simulink model "Wiper_System"  (R2018a)
settings: Solver=FixedStepDiscrete  StartTime=0.0  StopTime=10.0  FixedStep=0.01  RelTol=1e-3
settings Model: Creator=Choaib ELMADI  LastModifiedBy=Choaib ELMADI

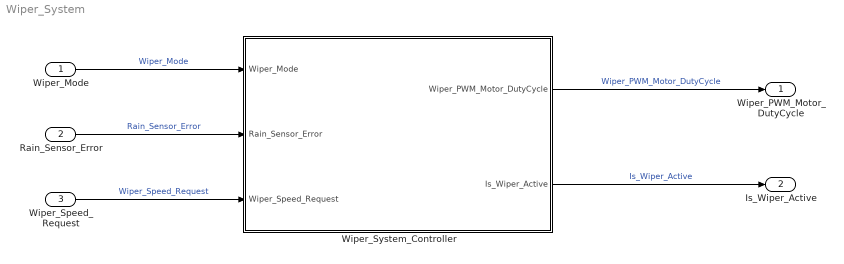
== system Wiper_System ==
  Wiper_Mode : Inport  OutMin=0  OutMax=3  OutDataTypeStr=double
  Rain_Sensor_Error : Inport  Port=2  OutMin=0  OutMax=1  OutDataTypeStr=double
  Wiper_Speed_Request : Inport  Port=3  OutMin=0  OutMax=7  OutDataTypeStr=double
  Wiper_System_Controller : Subsystem
  Wiper_PWM_Motor_DutyCycle : Outport  OutMin=0  OutMax=1  OutDataTypeStr=double
  Is_Wiper_Active : Outport  Port=2  OutMin=0  OutMax=1  OutDataTypeStr=double
  wires:
  Wiper_Mode/1 -> Wiper_System_Controller/1(Wiper_Mode)  "Wiper_Mode"
  Rain_Sensor_Error/1 -> Wiper_System_Controller/2(Rain_Sensor_Error)  "Rain_Sensor_Error"
  Wiper_Speed_Request/1 -> Wiper_System_Controller/3(Wiper_Speed_Request)  "Wiper_Speed_Request"
  Wiper_System_Controller/1(Wiper_PWM_Motor_DutyCycle) -> Wiper_PWM_Motor_DutyCycle/1  "Wiper_PWM_Motor_DutyCycle"
  Wiper_System_Controller/2(Is_Wiper_Active) -> Is_Wiper_Active/1  "Is_Wiper_Active"

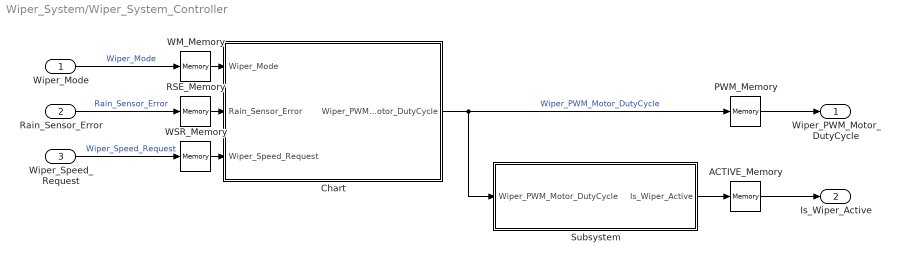
== system Wiper_System/Wiper_System_Controller ==
  Wiper_Mode : Inport
  Rain_Sensor_Error : Inport  Port=2
  Wiper_Speed_Request : Inport  Port=3
  ACTIVE_Memory : Memory
  Chart : Stateflow chart  TreatAsAtomicUnit=on
  PWM_Memory : Memory
  RSE_Memory : Memory
  Subsystem : Subsystem
  WM_Memory : Memory
  WSR_Memory : Memory
  Wiper_PWM_Motor_DutyCycle : Outport
  Is_Wiper_Active : Outport  Port=2
  wires:
  Wiper_Mode/1 -> WM_Memory/1  "Wiper_Mode"
  Rain_Sensor_Error/1 -> RSE_Memory/1  "Rain_Sensor_Error"
  Wiper_Speed_Request/1 -> WSR_Memory/1  "Wiper_Speed_Request"
  Chart/1(Wiper_PWM_Motor_DutyCycle) -> PWM_Memory/1, Subsystem/1(Wiper_PWM_Motor_DutyCycle)  "Wiper_PWM_Motor_DutyCycle"
  Subsystem/1(Is_Wiper_Active) -> ACTIVE_Memory/1
  WM_Memory/1 -> Chart/1(Wiper_Mode)
  RSE_Memory/1 -> Chart/2(Rain_Sensor_Error)
  WSR_Memory/1 -> Chart/3(Wiper_Speed_Request)
  PWM_Memory/1 -> Wiper_PWM_Motor_DutyCycle/1
  ACTIVE_Memory/1 -> Is_Wiper_Active/1

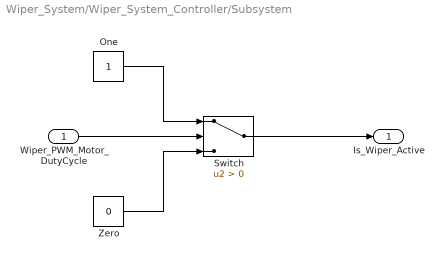
== system Wiper_System/Wiper_System_Controller/Subsystem ==
  Wiper_PWM_Motor_DutyCycle : Inport
  One : Constant
  Switch : Switch  Criteria=u2 > Threshold
  Zero : Constant  Value=0
  Is_Wiper_Active : Outport
  wires:
  Switch/1 -> Is_Wiper_Active/1
  Wiper_PWM_Motor_DutyCycle/1 -> Switch/2
  One/1 -> Switch/1
  Zero/1 -> Switch/3

== stateflow chart Wiper_System/Wiper_System_Controller/Chart ==
  state AUTO_MODE
    en:
    Wiper_PWM_Motor_DutyCycle = Wiper_Lookup_Table(Wiper_Speed_Request);
    du:
    Wiper_PWM_Motor_DutyCycle = Wiper_Lookup_Table(Wiper_Speed_Request);
  state OFF_MODE
    en:
    Wiper_PWM_Motor_DutyCycle = 0;
  state HIGH_SPEED_MODE
    en:
    Wiper_PWM_Motor_DutyCycle = 0.7;
  state LOW_SPEED_MODE
    en:
    Wiper_PWM_Motor_DutyCycle = 0.4;
  (default) -> OFF_MODE
  OFF_MODE -> (junction 23) : [Wiper_Mode ~= 0]
  AUTO_MODE -> (junction 23) : [Wiper_Mode ~= 1 || Rain_Sensor_Error  == 1]
  (junction 23) -> (junction 13)
  (junction 14) -> OFF_MODE [order 1] : [Wiper_Mode == 0 || (Wiper_Mode == 1 && Rain_Sensor_Error == 1)]
  (junction 18) -> AUTO_MODE [order 2] : [Wiper_Mode == 1 && Rain_Sensor_Error == 0]
  (junction 13) -> (junction 14) [order 1]
  (junction 13) -> (junction 18) [order 2]
  (junction 14) -> LOW_SPEED_MODE [order 2] : [Wiper_Mode == 2]
  (junction 24) -> (junction 13)
  (junction 18) -> HIGH_SPEED_MODE [order 1] : [Wiper_Mode == 3]
  LOW_SPEED_MODE -> (junction 24) : [Wiper_Mode ~= 2]
  HIGH_SPEED_MODE -> (junction 24) : [Wiper_Mode ~= 3]
  data: request function_input; speed function_output; Wiper_Mode input; Rain_Sensor_Error input; Wiper_Speed_Request input; Wiper_PWM_Motor_DutyCycle output
  function speed = Wiper_Lookup_Table(request):
    | function speed = Wiper_Lookup_Table(request)
    |     Wiper_Speed_Table = [0 0.4 0.45 0.5 0.55 0.6 0.65 0.7];
    |     speed = Wiper_Speed_Table(uint8(request + 1));
    | end
